simulink model "LQR1"  (R2020a)
settings: Solver=VariableStepAuto  StartTime=0.0  StopTime=10.0  RelTol=1e-3
settings Model: Creator=niran  LastModifiedBy=niran

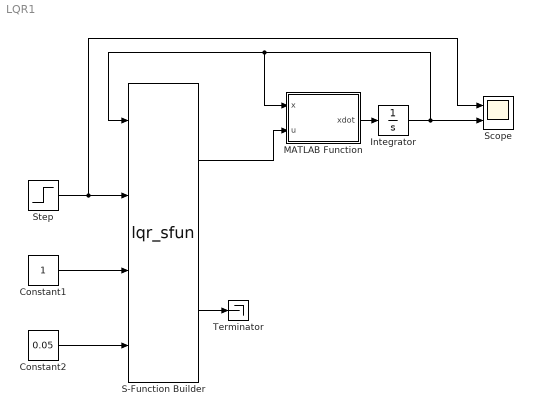
== system LQR1 ==
  Constant1 : Constant
  Constant2 : Constant  Value=0.05
  Integrator : Integrator
  MATLAB Function : MATLAB Function  TreatAsAtomicUnit=on
  S-Function Builder : S-Function  InitFcn=try, set_param(gcb,'FunctionName','lqr_sfun'), end  FunctionName=lqr_sfun  SFunctionModules=lqr_sfun_wrapper lqr_code lqr_code_Call  SFunctionDeploymentMode=off  EnableBusSupport=off  mask(S-Function Builder){}
      mask help: Simulink:masks:SFunctionBuilder_MD
      mask init:
      | val = [[.9  0.75 0.75 1 1 .9 .9 1]',[1 1 0.75 0.75 .9 .9 1 .9]'];try , sys = get_param(gcb,'SfunBuilderFcnName');if isempty(sys), sys = get_param(gcb,'FunctionName'); end,catch, sys = get_param(gcb,'FunctionName'); end
      settings: CopyFcn=set_param(gcbh,'LinkStatus','none')  PreSaveFcn=try, set_param(gcb,'FunctionName','lqr_sfun'), end  OpenFcn=sfunctionwizard(gcbh)
      mask Display: plot(val(:,1),val(:,2)),disp(sys), port_label('input',1,'x'), port_label('input',2,'ref'), port_label('input',3,'Q'), port_label('input',4,'R'), port_label('output',1,'u'), port_label('output',2,'K')
  Scope : Scope  NumInputPorts=2
  Step : Step  Time=5  Before=0.5  SampleTime=0
  Terminator : Terminator
  wires:
  MATLAB Function/1(xdot) -> Integrator/1
  Integrator/1 -> Scope/2, MATLAB Function/1(x), S-Function Builder/1
  S-Function Builder/1 -> MATLAB Function/2(u)
  S-Function Builder/2 -> Terminator/1
  Constant2/1 -> S-Function Builder/4
  Constant1/1 -> S-Function Builder/3
  Step/1 -> S-Function Builder/2, Scope/1

== matlab function LQR1/MATLAB Function ==
  data: x input; u input; xdot output
function xdot = fcn(x, u)

xdot = -x + u;
